simulink model "GFM_NN_closedloop"  (R2025a)
settings: Solver=FixedStepAuto  StartTime=0.0  StopTime=8  FixedStep=1e-6  RelTol=1e-5
PostLoadFcn:
  | , if any(exist('dsrtsu_mdlpostloadfcn', 'file') == [2, 3, 6]), try dsrtsu_mdlpostloadfcn('Execute', bdroot); catch fprintf('Error in PostLoadFcn (dsrtsu_mdlpostloadfcn) for model "%s":\n %s\n', bdroot, lasterr); end, end,
InitFcn:
  | %% ---------sampling time---------
  | fs=10000;
  | Ts = 1/fs; % 1/fs = sampling period;
  | Tsp=Ts;
  | ws=2*pi*fs;
  | Tc = Ts/1;
  | Tch = inf;
  | % Interrupt shift
  | %Tint=0.25e-6;
  | Tint=0.25e-6;
  | %Tint=0;
  | 
  | %% Frequency
  | fsw = 10e3;
  | Tsp = 1 / fsw;
  | % Ts = 1e-6;
  | 
  | %% Grid parameters
  | Vg_LG_RMS = 110;
  | Vg_LL_RMS = Vg_LG_RMS * sqrt(3);
  | f1 = 50;
  | w1 = f1 * 2 * pi;
  | 
  | Lg = 15e-3;
  | Rg = w1 * Lg * 0.05;
  | 
  | %% GFM converter
  | peak_phase_to_earth = sqrt(2)/sqrt(3);
  | SN_GFM = 4e3;
  | PN_GFM = SN_GFM;
  | Vtr_1 = 132;
  | V_base_GFL = Vtr_1*peak_phase_to_earth;
  | I_base_GFL = SN_GFM*peak_phase_to_earth/Vtr_1;
  | 
  | Vs_LL_RMS = Vg_LL_RMS;
  | VDC = 600;
  | 
  | Ls = 3e-3;
  | Rs = w1 * Ls * 0.05;
  | % Rs = 1e-1;
  | Cf = 10e-6;
  | Rf = 1e-3;
  | % Rf = 1;
  | 
  | %% Base values
  | w_Base = 1;
  | %w_Base = 2*pi*f1;
  | V_Base_GFM = sqrt(2) * Vs_LL_RMS / sqrt(3);      % Peak value
  | S_Base_GFM = SN_GFM;
  | I_Base_GFM = sqrt(2) * (S_Base_GFM / 3) / (V_Base_GFM / sqrt(2));     % Peak value
  | Z_Base_GFM = V_Base_GFM / I_Base_GFM;
  | L_Base_GFM = Z_Base_GFM / w_Base;
  | C_Base_GFM = 1 / (w_Base * Z_Base_GFM);
  | 
  | w1_pu = w1 / w_Base;
  | 
  | %% PU values
  | Ls * w1_pu / Z_Base_GFM
  | Ls_pu = Ls / Z_Base_GFM;
  | Lg_pu = Lg / Z_Base_GFM;
  | ... (+142 lines)
model workspace (MAT data in the model file):
  W1 = [0.530351698399 -0.46726077795 -0.189978018403 0.581505596638 -0.976636350155 0.285457074642 -0.344555467367 -0.823834598064 0.260987460613 -0.174824804068 0.166140690446 -2.19062757492 ... (5120 elements, 64x80)]
  W2 = [0.0236483272165 -0.12587569654 -3.47338819504 -0.292541116476 -0.164569035172 -0.37011295557 -0.0788608714938 -0.34808665514 -0.0821482911706 0.0780714154243 -0.721733689308 -0.485419809818 ... (1024 elements, 16x64)]
  W3 = [-0.129827529192 0.112917125225 -0.211720749736 0.109386667609 -1.40702748299 -1.11484694481 -0.318361610174 0.218052342534 0.374470740557 -0.190498560667 -0.238774597645 0.996348917484 ... (16 elements, 1x16)]
  b1 = [-8.9806804657 -10.8322944641 0.357735663652 -8.11319255829 -12.3089160919 -6.15159845352 -0.239361956716 -10.1425418854 -3.17705559731 -9.53854560852 -2.29398417473 -11.1701593399 ... (64 elements, 64x1)]
  b2 = [-0.136206507683 -0.45766967535 -1.54362010956 -0.556495547295 -0.369174063206 -1.49981951714 -1.85871458054 -0.587826907635 -4.87963867188 -1.14077246189 -0.44449698925 -0.9487388134 ... (16 elements, 16x1)]
  b3 = 2.70423817635
  iqrValues = [999.929682567 999.948806394 999.974126382 1163.68199033 1249.86143465 1016.10909761 999.955656405 999.968539404 999.977085124 999.966554003 999.979581889 999.988183479 ... (80 elements, 1x80)]
  medianValues = [1999.66013382 1999.76293028 1999.73262567 1999.76378275 1999.76361619 1999.77040731 1999.79192245 1999.85691047 1999.87382515 1999.88874694 1999.91524435 1999.91351393 ... (80 elements, 1x80)]
  mu = [-0.108593781339 -0.147308811259 -0.175534555128 -0.136585928467 -0.119784171193 -0.170883245612 -0.185899506459 -0.135931465846 -0.0891217813808 -0.0659545740614 -0.0558679902038 -0.052863332895 ... (80 elements, 1x80)]
  net2 : dlnetwork (value not decoded)
  sigma = [0.7187830922 0.834238393845 0.919900139685 0.688758980318 0.599693957155 0.858339742411 0.965167977116 0.792700626358 0.681503940515 0.658236278259 0.655707879722 0.655775233832 ... (80 elements, 1x80)]
undefined symbols (not defined in the file): DiscIntNeverNeededParam
libraries: spsSeriesRLCBranchLib x18, spsCurrentMeasurementLib x9, simulink x6, spsVoltageMeasurementLib x6, simulink_extras x4, spsGroundLib x4, plecslib_extras x2, deeplib x1, spsDCVoltageSourceLib x1, spsThreePhaseProgrammableVoltageSourceLib x1, spsTwoLevelConverterLib x1, spspowerguiLib x1
(part 2 of 3)

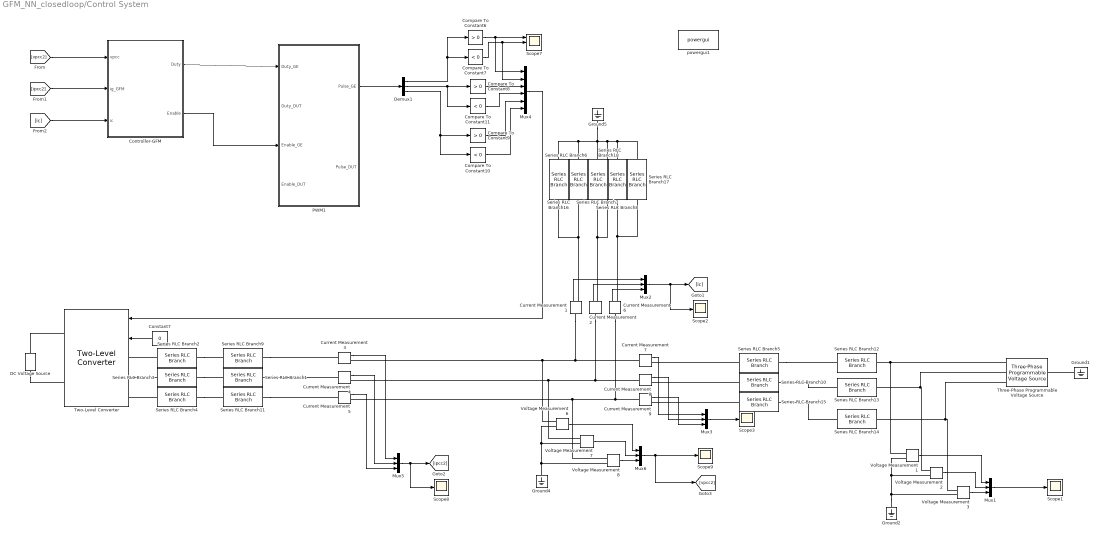
== system GFM_NN_closedloop/Control System ==
  Compare To Constant10 : simulink/Logic and Bit Operations/Compare To Constant  relop=<  const=0  OutDataTypeStr=uint8
  Compare To Constant11 : simulink/Logic and Bit Operations/Compare To Constant  relop=<  const=0  OutDataTypeStr=uint8
  Compare To Constant6 : simulink/Logic and Bit Operations/Compare To Constant  relop=>  const=0  OutDataTypeStr=uint8
  Compare To Constant7 : simulink/Logic and Bit Operations/Compare To Constant  relop=<  const=0  OutDataTypeStr=uint8
  Compare To Constant8 : simulink/Logic and Bit Operations/Compare To Constant  relop=>  const=0  OutDataTypeStr=uint8
  Compare To Constant9 : simulink/Logic and Bit Operations/Compare To Constant  relop=>  const=0  OutDataTypeStr=uint8
  Constant7 : Constant  Value=0
  Controller-GFM : Subsystem
  Current Measurement{1..9} (9 alike) : spsCurrentMeasurementLib/Current Measurement  PhasorSimulation=off  OutputType=Complex  PSBequivalent=0
  DC Voltage Source : spsDCVoltageSourceLib/DC Voltage Source  Amplitude=600  Measurements=None
  Demux1 : Demux  Outputs=3
  Ground{1..2,4..5} (4 alike) : spsGroundLib/Ground  LConnTagsString=a
  Mux{1..3,5..6} (5 alike) : Mux  Inputs=3
  Mux4 : Mux  Inputs=6
  PWM1 : Subsystem
  Scope{1..3,8..9} (5 alike) : Scope
      Scope1 settings: ActiveDisplayYMinimum=-125  ActiveDisplayYMaximum=125
      Scope2 settings: ActiveDisplayYMinimum=-50.45124  ActiveDisplayYMaximum=47.16333
      Scope3 settings: ActiveDisplayYMinimum=-17.02928  ActiveDisplayYMaximum=18.03944  DataLoggingVariableName=Ipcc_f
      Scope8 settings: ActiveDisplayYMinimum=-37.50909  ActiveDisplayYMaximum=37.34562  DataLoggingVariableName=Ipcc
      Scope9 settings: ActiveDisplayYMinimum=-922.38426  ActiveDisplayYMaximum=758.14145
  Scope7 : Scope  NumInputPorts=3
      settings: ActiveDisplayYMinimum=-0.03656  ActiveDisplayYMaximum=1.05589  DataLoggingVariableName=ScopeData2
  Series RLC Branch1 : spsSeriesRLCBranchLib/Series RLC Branch  LConnTagsString=__new0  RConnTagsString=__new0  BranchType=L  Resistance=0.5  Inductance=2e-3  SetiL0=off  InitialCurrent=0  Capacitance=1e-6  Setx0=off  InitialVoltage=0  Measurements=None
  Series RLC Branch{2..5,10,15} (6 alike) : spsSeriesRLCBranchLib/Series RLC Branch  LConnTagsString=__new0  RConnTagsString=__new0  BranchType=R  Resistance=0.2  Inductance=2e-3  SetiL0=off  InitialCurrent=0  Capacitance=1e-6  Setx0=off  InitialVoltage=0  Measurements=None
  Series RLC Branch11 : spsSeriesRLCBranchLib/Series RLC Branch  LConnTagsString=__new0  RConnTagsString=__new0  BranchType=L  Resistance=0.5  Inductance=2e-3  SetiL0=off  InitialCurrent=0  Capacitance=1e-6  Setx0=off  InitialVoltage=0  Measurements=None
  Series RLC Branch12 : spsSeriesRLCBranchLib/Series RLC Branch  LConnTagsString=__new0  RConnTagsString=__new0  BranchType=L  Resistance=0.5  Inductance=20e-3  SetiL0=off  InitialCurrent=0  Capacitance=1e-6  Setx0=off  InitialVoltage=0  Measurements=None
  Series RLC Branch13 : spsSeriesRLCBranchLib/Series RLC Branch  LConnTagsString=__new0  RConnTagsString=__new0  BranchType=L  Resistance=0.5  Inductance=20e-3  SetiL0=off  InitialCurrent=0  Capacitance=1e-6  Setx0=off  InitialVoltage=0  Measurements=None
  Series RLC Branch14 : spsSeriesRLCBranchLib/Series RLC Branch  LConnTagsString=__new0  RConnTagsString=__new0  BranchType=L  Resistance=0.5  Inductance=20e-3  SetiL0=off  InitialCurrent=0  Capacitance=1e-6  Setx0=off  InitialVoltage=0  Measurements=None
  Series RLC Branch16 : spsSeriesRLCBranchLib/Series RLC Branch  LConnTagsString=__new0  RConnTagsString=__new0  BranchType=R  Resistance=20  Inductance=2e-3  SetiL0=off  InitialCurrent=0  Capacitance=1e-6  Setx0=off  InitialVoltage=0  Measurements=None
  Series RLC Branch17 : spsSeriesRLCBranchLib/Series RLC Branch  LConnTagsString=__new0  RConnTagsString=__new0  BranchType=R  Resistance=20  Inductance=2e-3  SetiL0=off  InitialCurrent=0  Capacitance=1e-6  Setx0=off  InitialVoltage=0  Measurements=None
  Series RLC Branch18 : spsSeriesRLCBranchLib/Series RLC Branch  LConnTagsString=__new0  RConnTagsString=__new0  BranchType=R  Resistance=20  Inductance=2e-3  SetiL0=off  InitialCurrent=0  Capacitance=1e-6  Setx0=off  InitialVoltage=0  Measurements=None
  Series RLC Branch6 : spsSeriesRLCBranchLib/Series RLC Branch  LConnTagsString=__new0  RConnTagsString=__new0  BranchType=C  Resistance=0.5  Inductance=5e-3  SetiL0=off  InitialCurrent=0  Capacitance=10e-6  Setx0=off  InitialVoltage=0  Measurements=None
  Series RLC Branch7 : spsSeriesRLCBranchLib/Series RLC Branch  LConnTagsString=__new0  RConnTagsString=__new0  BranchType=C  Resistance=0.5  Inductance=5e-3  SetiL0=off  InitialCurrent=0  Capacitance=10e-6  Setx0=off  InitialVoltage=0  Measurements=None
  Series RLC Branch8 : spsSeriesRLCBranchLib/Series RLC Branch  LConnTagsString=__new0  RConnTagsString=__new0  BranchType=C  Resistance=0.5  Inductance=5e-3  SetiL0=off  InitialCurrent=0  Capacitance=10e-6  Setx0=off  InitialVoltage=0  Measurements=None
  Series RLC Branch9 : spsSeriesRLCBranchLib/Series RLC Branch  LConnTagsString=__new0  RConnTagsString=__new0  BranchType=L  Resistance=0.5  Inductance=2e-3  SetiL0=off  InitialCurrent=0  Capacitance=1e-6  Setx0=off  InitialVoltage=0  Measurements=None
  Three-Phase Programmable Voltage Source : spsThreePhaseProgrammableVoltageSourceLib/Three-Phase Programmable Voltage Source  PositiveSequence="[100*sqrt(3)/sqrt(2)  0 50]"  VariationEntity=Amplitude  VariationType=Table of time-amplitude pairs  VariationTypeAlt=Step  VariationStep=0.5  VariationRate=10  VariationMagnitude=0.3  VariationFrequency=2  VariationTiming=[1 2]  VariationPhaseA=off  Amplitudes=[1 0.5]  TimeValues=[0 5]  HarmonicGeneration=off  HarmonicA=[3 0.2 -25 0]  HarmonicB=[2 0.15 35 2]  Timing="[0.05  3]"  BusType=swing  Pref=0  Qref=0  Qmin=-inf  Qmax=inf
  Two-Level Converter : spsTwoLevelConverterLib/Two-Level Converter  ModelType=Switching devices  Ron=1e-3  Rs=1e6  Cs=inf  Vforward=[0,0]  Ron_Diode=1e-3  Rs_Diode=1e6  Cs_Diode=inf  Vf_Diode=1e-3  Rs_CurrentSource=inf  Ron_ACsource=1e-3
      settings: LibrarySourceBlock=sps_lib/Power Electronics/Two-Level Converter
  Voltage Measurement{1..3,6..8} (6 alike) : spsVoltageMeasurementLib/Voltage Measurement  PhasorSimulation=off  OutputType=Complex  PSBequivalent=0
  powergui1 : spspowerguiLib/powergui  Priority=1  SimulationMode=Discrete  SampleTime=1e-6  frequency=60  Iterations=50  frequencyindice=0  Pbase=100e6  ErrMax=1e-4  UnitsV=kV  UnitsW=MW  buscounter=0  FunctionMessages=off  echomessages=off  EnableUseOfTLC=off  CurrentSourceSwitches=off  DisableSnubberDevices=off  DisableRonSwitches=off  DisableVfSwitches=off  DisplayEquations=off  AutomaticDiscreteSolvers=off  SolverType=Tustin/Backward Euler (TBE)  Interpol=off  ExternalGateDelay=off  methode=off  Ts=100  x0status=blocks  SPID=on  SwTol=0  HookPort=off  NonlinearTolerance=1e-4  nMaxIteration=100  ContinueOnMaxIteration=off  RestoreLinks=warning  ResistiveCurrentMeasurement=off  Frange=[0:2:500]  Ylog=off  Xlog=on  ShowGrid=off  save=off  variable=ZData  structure=0  ZoomFFT=off  StartTime=0.0  cycles=1  DisplayStyle=1  fundamental=60  FreqAxis=off  MaxFrequency=1000  frequencyindicesteady=1  RmsSteady=1  display=off
  wires:
  Mux4/1 -> Two-Level Converter/1
  Constant7/1 -> Two-Level Converter/2
  Compare To Constant7/1 -> Mux4/2, Scope7/2
  PWM1/1(Pulse_GE) -> Demux1/1
  Compare To Constant9/1 -> Mux4/5
  Compare To Constant11/1 -> Mux4/4
  Compare To Constant6/1 -> Scope7/1, Mux4/1
  Demux1/3 -> Compare To Constant10/1, Compare To Constant9/1
  Demux1/1 -> Compare To Constant7/1, Compare To Constant6/1
  Compare To Constant8/1 -> Mux4/3
  Demux1/2 -> Compare To Constant11/1, Compare To Constant8/1
  Compare To Constant10/1 -> Mux4/6
  Current Measurement3/1 -> Mux5/1
  Current Measurement4/1 -> Mux5/2
  Current Measurement5/1 -> Mux5/3
  Voltage Measurement7/1 -> Mux6/2
  Voltage Measurement6/1 -> Mux6/1
  Mux6/1 -> [vpcc2], Scope9/1
  Voltage Measurement8/1 -> Mux6/3
  Current Measurement7/1 -> Mux3/1
  Current Measurement8/1 -> Mux3/2
  Current Measurement9/1 -> Mux3/3
  Mux3/1 -> Scope3/1
  Mux5/1 -> Scope8/1, [ipcc2]
  Mux1/1 -> Scope1/1
  Voltage Measurement3/1 -> Mux1/3
  Voltage Measurement1/1 -> Mux1/1
  Voltage Measurement2/1 -> Mux1/2
  [vpcc2] -> Controller-GFM/1(vpcc)
  [ipcc2] -> Controller-GFM/2(ig_GFM)
  Controller-GFM/1(Duty) -> PWM1/1(Duty_GE)
  Controller-GFM/2(Enable) -> PWM1/3(Enable_GE)
  Current Measurement1/1 -> Mux2/1
  Current Measurement2/1 -> Mux2/2
  Current Measurement6/1 -> Mux2/3
  Mux2/1 -> Scope2/1, [ic]
  [ic] -> Controller-GFM/3(ic)
  connections:
  DC Voltage Source/RConn1 -- Two-Level Converter/RConn1
  DC Voltage Source/LConn1 -- Two-Level Converter/RConn2
  Series RLC Branch11/RConn1 -- Current Measurement5/LConn1
  Series RLC Branch1/RConn1 -- Current Measurement4/LConn1
  Series RLC Branch9/RConn1 -- Current Measurement3/LConn1
  Voltage Measurement7/LConn2 -- Voltage Measurement6/LConn2 -- Voltage Measurement8/LConn2 -- Ground4/LConn1
  Voltage Measurement7/LConn1 -- Current Measurement2/LConn1 -- Current Measurement8/LConn1 -- Current Measurement4/RConn1
  Series RLC Branch6/LConn1 -- Series RLC Branch16/LConn1 -- Series RLC Branch17/LConn1 -- Series RLC Branch8/LConn1 -- Series RLC Branch18/LConn1 -- Ground5/LConn1 -- Series RLC Branch7/LConn1
  Current Measurement3/RConn1 -- Current Measurement1/LConn1 -- Current Measurement7/LConn1 -- Voltage Measurement6/LConn1
  Current Measurement5/RConn1 -- Current Measurement6/LConn1 -- Current Measurement9/LConn1 -- Voltage Measurement8/LConn1
  Voltage Measurement1/LConn1 -- Series RLC Branch12/RConn1 -- Three-Phase Programmable Voltage Source/RConn1
  Voltage Measurement2/LConn1 -- Three-Phase Programmable Voltage Source/RConn2 -- Series RLC Branch13/RConn1
  Voltage Measurement3/LConn1 -- Three-Phase Programmable Voltage Source/RConn3 -- Series RLC Branch14/RConn1
  Ground1/LConn1 -- Three-Phase Programmable Voltage Source/LConn1
  Ground2/LConn1 -- Voltage Measurement3/LConn2 -- Voltage Measurement2/LConn2 -- Voltage Measurement1/LConn2
  Series RLC Branch2/LConn1 -- Two-Level Converter/LConn1
  Series RLC Branch2/RConn1 -- Series RLC Branch9/LConn1
  Series RLC Branch3/LConn1 -- Two-Level Converter/LConn2
  Series RLC Branch3/RConn1 -- Series RLC Branch1/LConn1
  Series RLC Branch4/LConn1 -- Two-Level Converter/LConn3
  Series RLC Branch4/RConn1 -- Series RLC Branch11/LConn1
  Series RLC Branch5/RConn1 -- Series RLC Branch12/LConn1
  Series RLC Branch5/LConn1 -- Current Measurement7/RConn1
  Series RLC Branch10/LConn1 -- Current Measurement8/RConn1
  Series RLC Branch10/RConn1 -- Series RLC Branch13/LConn1
  Series RLC Branch15/LConn1 -- Current Measurement9/RConn1
  Series RLC Branch15/RConn1 -- Series RLC Branch14/LConn1
  Current Measurement1/RConn1 -- Series RLC Branch16/RConn1 -- Series RLC Branch6/RConn1
  Series RLC Branch7/RConn1 -- Series RLC Branch18/RConn1 -- Current Measurement2/RConn1
  Series RLC Branch8/RConn1 -- Series RLC Branch17/RConn1 -- Current Measurement6/RConn1

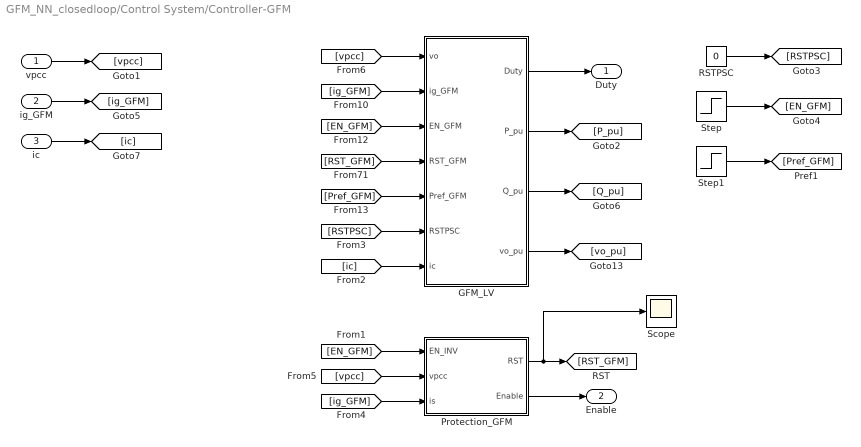
== system GFM_NN_closedloop/Control System/Controller-GFM ==
  vpcc : Inport
  ig_GFM : Inport  Port=2
  ic : Inport  Port=3
  GFM_LV : Subsystem
  Protection_GFM : Subsystem
  RSTPSC : Constant  Value=0
  Scope : Scope
      settings: ActiveDisplayYMinimum=-0.125  ActiveDisplayYMaximum=1.125  DataLoggingVariableName=ScopeData3
  Step : Step  Time=0.5  SampleTime=0
  Step1 : Step  Time=3  After=1500  SampleTime=0
  Duty : Outport  VectorParamsAs1DForOutWhenUnconnected=off
  Enable : Outport  Port=2  VectorParamsAs1DForOutWhenUnconnected=off
  wires:
  vpcc/1 -> [vpcc]
  ig_GFM/1 -> [ig_GFM]
  [vpcc] -> GFM_LV/1(vo)
  [ig_GFM] -> GFM_LV/2(ig_GFM)
  [EN_GFM] -> GFM_LV/3(EN_GFM)
  [Pref_GFM] -> GFM_LV/5(Pref_GFM)
  GFM_LV/2(P_pu) -> [P_pu]
  GFM_LV/3(Q_pu) -> [Q_pu]
  GFM_LV/1(Duty) -> Duty/1
  [EN_GFM] -> Protection_GFM/1(EN_INV)
  Protection_GFM/1(RST) -> Scope/1, [RST_GFM]
  Protection_GFM/2(Enable) -> Enable/1
  [ig_GFM] -> Protection_GFM/3(is)
  [vpcc] -> Protection_GFM/2(vpcc)
  Step/1 -> [EN_GFM]
  RSTPSC/1 -> [RSTPSC]
  Step1/1 -> [Pref_GFM]
  GFM_LV/4(vo_pu) -> [vo_pu]
  [RSTPSC] -> GFM_LV/6(RSTPSC)
  [RST_GFM] -> GFM_LV/4(RST_GFM)
  ic/1 -> [ic]
  [ic] -> GFM_LV/7(ic)

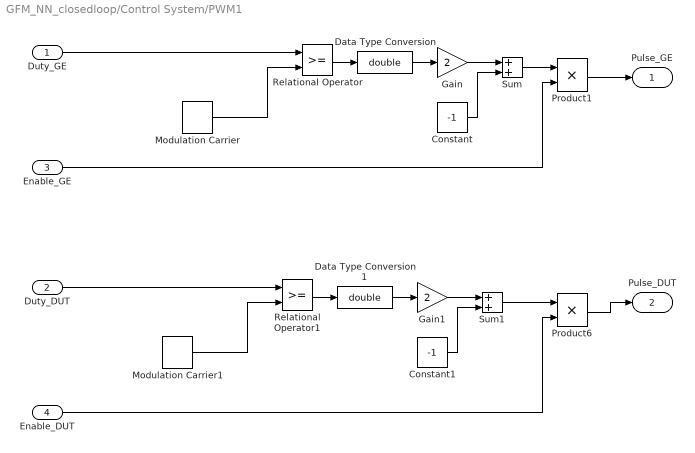
== system GFM_NN_closedloop/Control System/PWM1 ==
  Duty_GE : Inport
  Duty_DUT : Inport  Port=2
  Enable_GE : Inport  Port=3
  Enable_DUT : Inport  Port=4
  Constant : Constant  Value=-1  SampleTime=-1
  Constant1 : Constant  Value=-1  SampleTime=-1
  Data Type Conversion : DataTypeConversion  OutDataTypeStr=double
  Data Type Conversion1 : DataTypeConversion  OutDataTypeStr=double
  Gain : Gain  Gain=2  SaturateOnIntegerOverflow=on  OutDataTypeStr=Inherit: Same as input  ParamDataTypeStr=Inherit: Same as input
  Gain1 : Gain  Gain=2  SaturateOnIntegerOverflow=on  OutDataTypeStr=Inherit: Same as input  ParamDataTypeStr=Inherit: Same as input
  Modulation Carrier : plecslib_extras/Modulators/Symmetrical PWM/Modulation Carrier  fc=10e3  offset=mod(0.5, 1)  range=[0 1]
  Modulation Carrier1 : plecslib_extras/Modulators/Symmetrical PWM/Modulation Carrier  fc=10e3  offset=mod(0.5, 1)  range=[0 1]
  Product1 : Product
  Product6 : Product
  Relational Operator : RelationalOperator
  Relational Operator1 : RelationalOperator
  Sum : Sum  InputSameDT=on  SaturateOnIntegerOverflow=on  OutDataTypeStr=Inherit: Same as first input
  Sum1 : Sum  InputSameDT=on  SaturateOnIntegerOverflow=on  OutDataTypeStr=Inherit: Same as first input
  Pulse_GE : Outport  VectorParamsAs1DForOutWhenUnconnected=off
  Pulse_DUT : Outport  Port=2  VectorParamsAs1DForOutWhenUnconnected=off
  wires:
  Duty_GE/1 -> Relational Operator/1
  Modulation Carrier/1 -> Relational Operator/2
  Relational Operator/1 -> Data Type Conversion/1
  Gain/1 -> Sum/1
  Constant/1 -> Sum/2
  Data Type Conversion/1 -> Gain/1
  Data Type Conversion1/1 -> Gain1/1
  Constant1/1 -> Sum1/2
  Gain1/1 -> Sum1/1
  Relational Operator1/1 -> Data Type Conversion1/1
  Modulation Carrier1/1 -> Relational Operator1/2
  Duty_DUT/1 -> Relational Operator1/1
  Sum1/1 -> Product6/1
  Product6/1 -> Pulse_DUT/1
  Enable_DUT/1 -> Product6/2
  Sum/1 -> Product1/1
  Product1/1 -> Pulse_GE/1
  Enable_GE/1 -> Product1/2

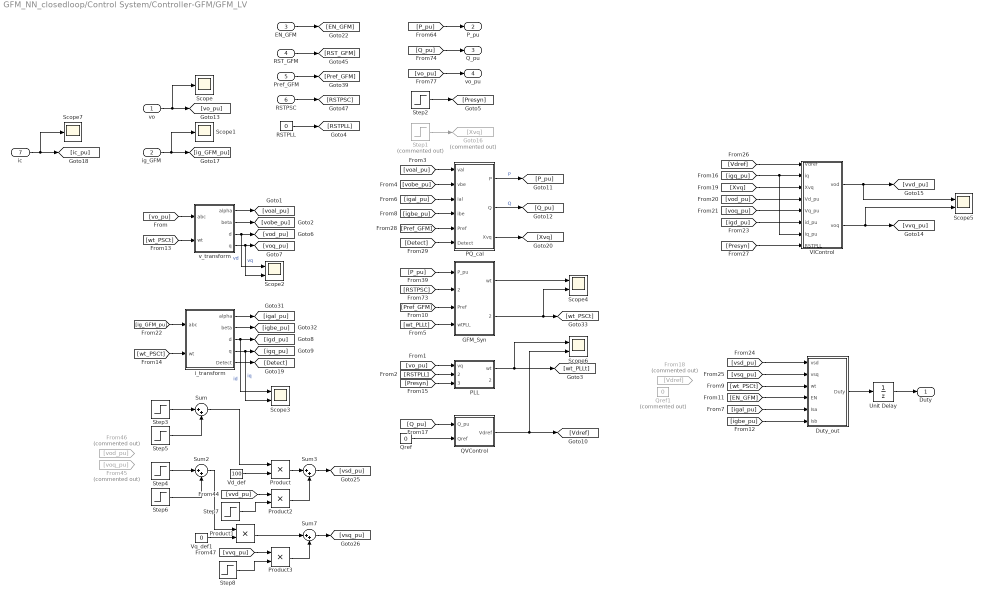
== system GFM_NN_closedloop/Control System/Controller-GFM/GFM_LV ==
  vo : Inport
  ig_GFM : Inport  Port=2
  EN_GFM : Inport  Port=3
  RST_GFM : Inport  Port=4
  Pref_GFM : Inport  Port=5
  RSTPSC : Inport  Port=6
  ic : Inport  Port=7
  Duty_out : Subsystem
  From18 : From  Commented=on  GotoTag=Vdref
  From45 : From  Commented=on  GotoTag=voq_pu
  From46 : From  Commented=on  GotoTag=vod_pu
  GFM_Syn : Subsystem
  Goto16 : Goto  Commented=on  GotoTag=Xvq
  PLL : Subsystem
  PQ_cal : Subsystem
  Product{,1..3} (4 alike) : Product
  QVControl : Subsystem
  Qref : Constant  Value=0
  Qref1 : Constant  Commented=on  Value=0
  RSTPLL : Constant  Value=0
  Scope : Scope
      settings: ActiveDisplayYMinimum=-224.40301  ActiveDisplayYMaximum=188.39301  DataLoggingVariableName=ScopeData4
  Scope1 : Scope
      settings: ActiveDisplayYMinimum=-5.9317  ActiveDisplayYMaximum=5.05503  DataLoggingVariableName=ScopeData5
  Scope{2..6} (5 alike) : Scope  NumInputPorts=2
      Scope2 settings: ActiveDisplayYMinimum=-686.32564  ActiveDisplayYMaximum=654.29928  DataLoggingVariableName=ScopeData9
      Scope3 settings: ActiveDisplayYMinimum=-36.80832  ActiveDisplayYMaximum=81.95422  DataLoggingVariableName=ScopeData10
      Scope4 settings: ActiveDisplayYMinimum=-592.09969  ActiveDisplayYMaximum=5328.89724  DataLoggingVariableName=ScopeData4
      Scope5 settings: ActiveDisplayYMinimum=-140.77704  ActiveDisplayYMaximum=348.97523
      Scope6 settings: ActiveDisplayYMinimum=-35.97431  ActiveDisplayYMaximum=302.6074  DataLoggingVariableName=ScopeData2
  Scope7 : Scope
      settings: ActiveDisplayYMinimum=-5.9317  ActiveDisplayYMaximum=5.05503  DataLoggingVariableName=ScopeData2
  Step1 : Step  Commented=on  Time=5.2  After=0  SampleTime=0
  Step2 : Step  Before=1  After=0  SampleTime=0
  Step3 : Step  Time=1.5  Before=1  After=0.5  SampleTime=0
  Step4 : Step  Time=1.5  Before=1  After=0.5  SampleTime=0
  Step5 : Step  Time=2  After=-0.5  SampleTime=0
  Step6 : Step  Time=2  After=-0.5  SampleTime=0
  Step7 : Step  Time=1.2  SampleTime=0
  Step8 : Step  Time=1.2  SampleTime=0
  Sum{,2..3,7} (4 alike) : Sum  Inputs=|++
  Unit Delay : UnitDelay  SampleTime=Ts  HasFrameUpgradeWarning=on
  VIControl : Subsystem
  Vd_def : Constant  Value=100
  Vq_def1 : Constant  Value=0
  i_transform : Subsystem
  v_transform : Subsystem
  Duty : Outport
  P_pu : Outport  Port=2
  Q_pu : Outport  Port=3
  vo_pu : Outport  Port=4
  wires:
  [voal_pu] -> PQ_cal/1(val)
  [vobe_pu] -> PQ_cal/2(vbe)
  [igal_pu] -> PQ_cal/3(ial)
  [igbe_pu] -> PQ_cal/4(ibe)
  PQ_cal/1(P) -> [P_pu]  "P"
  PQ_cal/2(Q) -> [Q_pu]  "Q"
  EN_GFM/1 -> [EN_GFM]
  [wt_PSCt] -> i_transform/2(wt)
  [ig_GFM_pu] -> i_transform/1(abc)
  [vo_pu] -> v_transform/1(abc)
  [wt_PSCt] -> v_transform/2(wt)
  v_transform/1(alpha) -> [voal_pu]
  [wt_PSCt] -> Duty_out/3(wt)
  [EN_GFM] -> Duty_out/4(EN)
  i_transform/1(alpha) -> [igal_pu]
  i_transform/2(beta) -> [igbe_pu]
  GFM_Syn/1(wt) -> Scope4/1
  [P_pu] -> GFM_Syn/1(P_pu)
  GFM_Syn/2(wtmod) -> Scope4/2, [wt_PSCt]
  RST_GFM/1 -> [RST_GFM]
  [RSTPSC] -> GFM_Syn/2(RSTPSC)
  Pref_GFM/1 -> [Pref_GFM]
  [P_pu] -> P_pu/1
  [Q_pu] -> Q_pu/1
  [vo_pu] -> vo_pu/1
  RSTPSC/1 -> [RSTPSC]
  v_transform/2(beta) -> [vobe_pu]
  [Pref_GFM] -> GFM_Syn/3(Pref)
  Duty_out/1(Duty) -> Unit Delay/1
  Unit Delay/1 -> Duty/1
  [igal_pu] -> Duty_out/5(Isa)
  [igbe_pu] -> Duty_out/6(Isb)
  [RSTPLL] -> PLL/2(RSTPLL)
  [vo_pu] -> PLL/1(vq)
  RSTPLL/1 -> [RSTPLL]
  [wt_PLLt] -> GFM_Syn/4(wtPLL)
  Step2/1 -> [Presyn]
  [Presyn] -> PLL/3(Presyn)
  vo/1 -> Scope/1, [vo_pu]
  ig_GFM/1 -> Scope1/1, [ig_GFM_pu]
  v_transform/3(d) -> Scope2/1, [vod_pu]  "vd"
  v_transform/4(q) -> Scope2/2, [voq_pu]  "vq"
  i_transform/3(d) -> Scope3/1, [igd_pu]  "id"
  i_transform/4(q) -> Scope3/2, [igq_pu]  "iq"
  [Q_pu] -> QVControl/1(Q_pu)
  QVControl/1(Vdref) -> Scope6/2, [Vdref]
  Qref/1 -> QVControl/2(Qref)
  [igq_pu] -> VIControl/7(iq_pu), VIControl/2(iq)
  [Xvq] -> VIControl/3(Xvq)
  [vod_pu] -> VIControl/4(Vd_pu)
  [voq_pu] -> VIControl/5(Vq_pu)
  [igd_pu] -> VIControl/6(id_pu)
  Step1/1 -> Goto16/1
  [Vdref] -> VIControl/1(Vdref)
  PLL/1(wt) -> Scope6/1, [wt_PLLt]
  [Presyn] -> VIControl/8(RSTPLL)
  [vsd_pu] -> Duty_out/1(vsd)
  [vsq_pu] -> Duty_out/2(vsq)
  Step6/1 -> Sum2/2
  Sum2/1 -> Product1/1
  Product1/1 -> Sum7/1
  Step5/1 -> Sum/2
  Product/1 -> Sum3/1
  Sum3/1 -> [vsd_pu]
  Sum/1 -> Product/1
  Step4/1 -> Sum2/1
  Sum7/1 -> [vsq_pu]
  Step3/1 -> Sum/1
  ic/1 -> Scope7/1, [ic_pu]
  VIControl/1(vod) -> [vvd_pu], Scope5/1
  VIControl/2(voq) -> [vvq_pu], Scope5/2
  [Pref_GFM] -> PQ_cal/5(Pref)
  i_transform/5(Detect) -> [Detect]
  [Detect] -> PQ_cal/6(Detect)
  PQ_cal/3(Xvq) -> [Xvq]
  [vvd_pu] -> Product2/1
  Product2/1 -> Sum3/2
  Step7/1 -> Product2/2
  Product3/1 -> Sum7/2
  [vvq_pu] -> Product3/1
  Step8/1 -> Product3/2
  Vd_def/1 -> Product/2
  Vq_def1/1 -> Product1/2

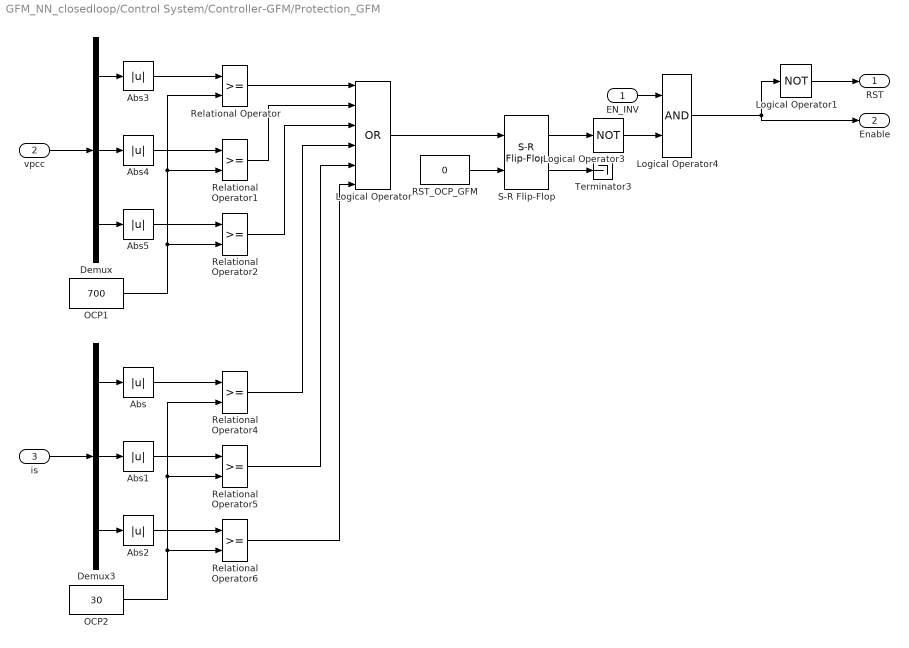
== system GFM_NN_closedloop/Control System/Controller-GFM/Protection_GFM ==
  EN_INV : Inport
  vpcc : Inport  Port=2
  is : Inport  Port=3
  Abs{,1..5} (6 alike) : Abs  SaturateOnIntegerOverflow=off
  Demux : Demux  Outputs=3
  Demux3 : Demux  Outputs=3
  Logical Operator : Logic  Operator=OR  Inputs=6  AllPortsSameDT=off  OutDataTypeStr=boolean
  Logical Operator1 : Logic  Operator=NOT  Inputs=1  IconShape=distinctive  AllPortsSameDT=off  OutDataTypeStr=boolean
  Logical Operator3 : Logic  Operator=NOT  Inputs=1  IconShape=distinctive  AllPortsSameDT=off  OutDataTypeStr=boolean
  Logical Operator4 : Logic  AllPortsSameDT=off  OutDataTypeStr=boolean
  OCP1 : Constant  Value=700
  OCP2 : Constant  Value=30
  RST_OCP_GFM : Constant  Value=0  OutDataTypeStr=boolean  SampleTime=-1
  Relational Operator{,1..2,4..6} (6 alike) : RelationalOperator  OutDataTypeStr=boolean  InputSameDT=off
  S-R Flip-Flop : simulink_extras/Flip Flops/S-R Flip-Flop  initial_condition=0
  Terminator3 : Terminator
  RST : Outport
  Enable : Outport  Port=2
  wires:
  Logical Operator1/1 -> RST/1
  Relational Operator/1 -> Logical Operator/1
  S-R Flip-Flop/1 -> Logical Operator3/1
  Relational Operator2/1 -> Logical Operator/3
  OCP2/1 -> Relational Operator6/2, Relational Operator5/2, Relational Operator4/2
  Relational Operator4/1 -> Logical Operator/4
  Logical Operator3/1 -> Logical Operator4/2
  Relational Operator5/1 -> Logical Operator/5
  Demux/1 -> Abs3/1
  OCP1/1 -> Relational Operator/2, Relational Operator1/2, Relational Operator2/2
  Relational Operator6/1 -> Logical Operator/6
  Demux/2 -> Abs4/1
  RST_OCP_GFM/1 -> S-R Flip-Flop/2
  Demux/3 -> Abs5/1
  S-R Flip-Flop/2 -> Terminator3/1
  Logical Operator/1 -> S-R Flip-Flop/1
  Demux3/1 -> Abs/1
  Demux3/2 -> Abs1/1
  EN_INV/1 -> Logical Operator4/1
  Abs4/1 -> Relational Operator1/1
  Relational Operator1/1 -> Logical Operator/2
  Abs1/1 -> Relational Operator5/1
  Abs3/1 -> Relational Operator/1
  Demux3/3 -> Abs2/1
  Abs/1 -> Relational Operator4/1
  Logical Operator4/1 -> Logical Operator1/1, Enable/1
  Abs2/1 -> Relational Operator6/1
  Abs5/1 -> Relational Operator2/1
  vpcc/1 -> Demux/1
  is/1 -> Demux3/1

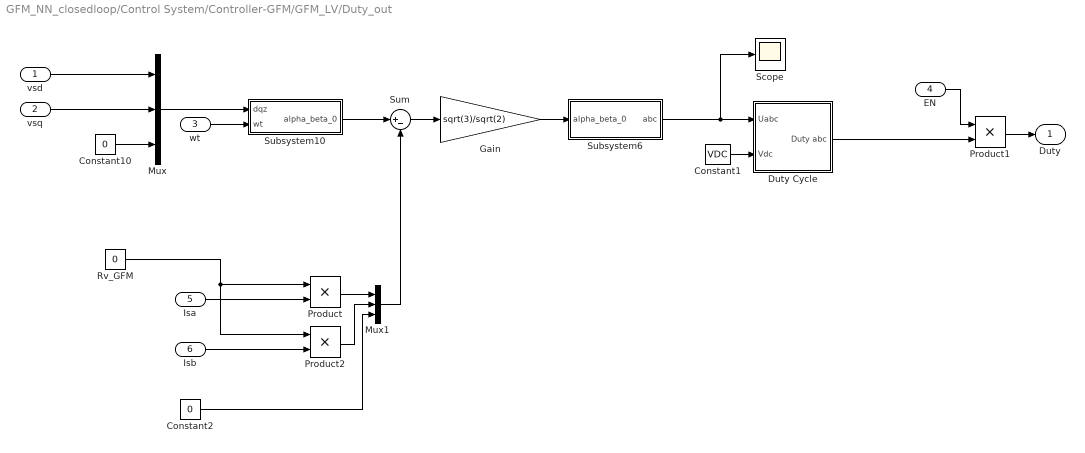
== system GFM_NN_closedloop/Control System/Controller-GFM/GFM_LV/Duty_out ==
  vsd : Inport
  vsq : Inport  Port=2
  wt : Inport  Port=3
  EN : Inport  Port=4
  Isa : Inport  Port=5
  Isb : Inport  Port=6
  Constant1 : Constant  Value=VDC
  Constant10 : Constant  Value=0
  Constant2 : Constant  Value=0
  Duty Cycle : Subsystem
  Gain : Gain  Gain=sqrt(3)/sqrt(2)
  Mux : Mux  Inputs=3
  Mux1 : Mux  Inputs=3
  Product : Product
  Product1 : Product
  Product2 : Product
  Rv_GFM : Constant  Value=0
  Scope : Scope
      settings: ActiveDisplayYMinimum=-202.9779  ActiveDisplayYMaximum=184.85798  DataLoggingVariableName=ScopeData7
  Subsystem10 : Subsystem
  Subsystem6 : Subsystem
  Sum : Sum  Inputs=|+-
  Duty : Outport
  wires:
  Product1/1 -> Duty/1
  Constant10/1 -> Mux/3
  EN/1 -> Product1/1
  Subsystem6/1(abc) -> Scope/1, Duty Cycle/1(Uabc)
  Constant1/1 -> Duty Cycle/2(Vdc)
  Mux/1 -> Subsystem10/1(dqz)
  wt/1 -> Subsystem10/2(wt)
  vsd/1 -> Mux/1
  vsq/1 -> Mux/2
  Duty Cycle/1(Duty abc) -> Product1/2
  Isa/1 -> Product/2
  Isb/1 -> Product2/2
  Rv_GFM/1 -> Product2/1, Product/1
  Subsystem10/1(alpha_beta_0) -> Sum/1
  Product/1 -> Mux1/1
  Product2/1 -> Mux1/2
  Mux1/1 -> Sum/2
  Constant2/1 -> Mux1/3
  Sum/1 -> Gain/1
  Gain/1 -> Subsystem6/1(alpha_beta_0)

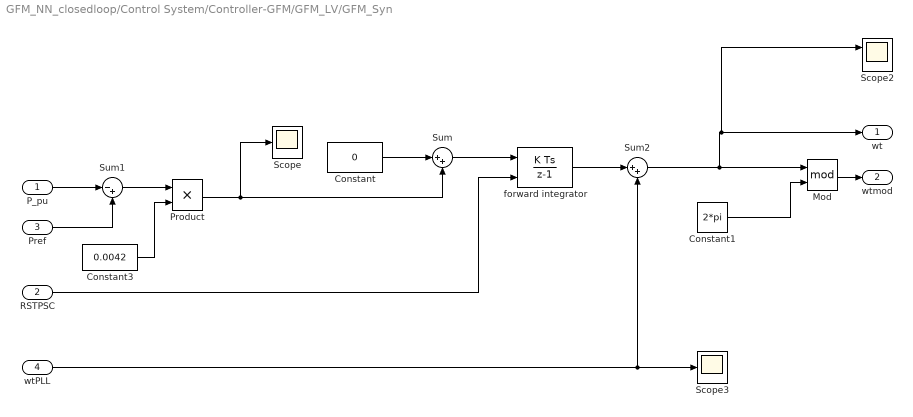
== system GFM_NN_closedloop/Control System/Controller-GFM/GFM_LV/GFM_Syn ==
  P_pu : Inport
  RSTPSC : Inport  Port=2
  Pref : Inport  Port=3
  wtPLL : Inport  Port=4
  Constant : Constant  Value=0
  Constant1 : Constant  Value=2*pi
  Constant3 : Constant  Value=0.0042
  Mod : Math  Operator=mod  SignedPower=on
  Product : Product
  Scope : Scope
      settings: ActiveDisplayYMinimum=-221.44913  ActiveDisplayYMaximum=185.90627  DataLoggingVariableName=ScopeData6
  Scope2 : Scope  NumInputPorts=2
      settings: ActiveDisplayYMinimum=-589.33689  ActiveDisplayYMaximum=5299.63804
  Scope3 : Scope
      settings: ActiveDisplayYMinimum=-51.78258  ActiveDisplayYMaximum=48.72639  DataLoggingVariableName=ScopeData3
  Sum : Sum  Inputs=|++
  Sum1 : Sum  Inputs=|-+
  Sum2 : Sum  Inputs=|++
  forward integrator : DiscreteIntegrator  ExternalReset=level  SampleTime=-1  ICPrevOutput=DiscIntNeverNeededParam  ICPrevScaledInput=DiscIntNeverNeededParam
  wt : Outport
  wtmod : Outport  Port=2
  wires:
  Constant/1 -> Sum/1
  Constant1/1 -> Mod/2
  Mod/1 -> wtmod/1
  Pref/1 -> Sum1/2
  Sum1/1 -> Product/1
  Product/1 -> Sum/2, Scope/1
  Sum/1 -> forward integrator/1
  forward integrator/1 -> Sum2/1
  wtPLL/1 -> Sum2/2, Scope3/1
  Sum2/1 -> Scope2/1, wt/1, Mod/1
  Constant3/1 -> Product/2
  RSTPSC/1 -> forward integrator/2
  P_pu/1 -> Sum1/1

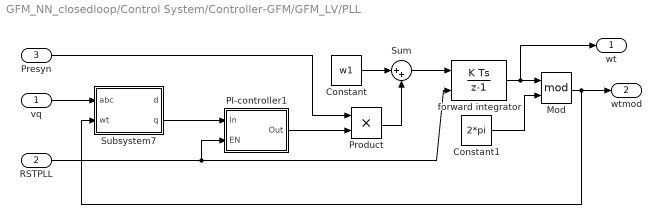
== system GFM_NN_closedloop/Control System/Controller-GFM/GFM_LV/PLL ==
  vq : Inport
  RSTPLL : Inport  Port=2
  Presyn : Inport  Port=3
  Constant : Constant  Value=w1
  Constant1 : Constant  Value=2*pi
  Mod : Math  Operator=mod  SignedPower=on
  PI-controller1 : Subsystem
      mask Display: disp('PI')
  Product : Product
  Subsystem7 : Subsystem
  Sum : Sum  Inputs=|++
  forward integrator : DiscreteIntegrator  ExternalReset=level  SampleTime=-1  ICPrevOutput=DiscIntNeverNeededParam  ICPrevScaledInput=DiscIntNeverNeededParam
  wt : Outport
  wtmod : Outport  Port=2
  wires:
  RSTPLL/1 -> forward integrator/2, PI-controller1/2(EN)
  Sum/1 -> forward integrator/1
  forward integrator/1 -> wt/1, Mod/1
  Constant1/1 -> Mod/2
  Mod/1 -> wtmod/1, Subsystem7/2(wt)
  vq/1 -> Subsystem7/1(abc)
  PI-controller1/1(Out) -> Product/2
  Subsystem7/2(q) -> PI-controller1/1(In)
  Presyn/1 -> Product/1
  Product/1 -> Sum/2
  Constant/1 -> Sum/1

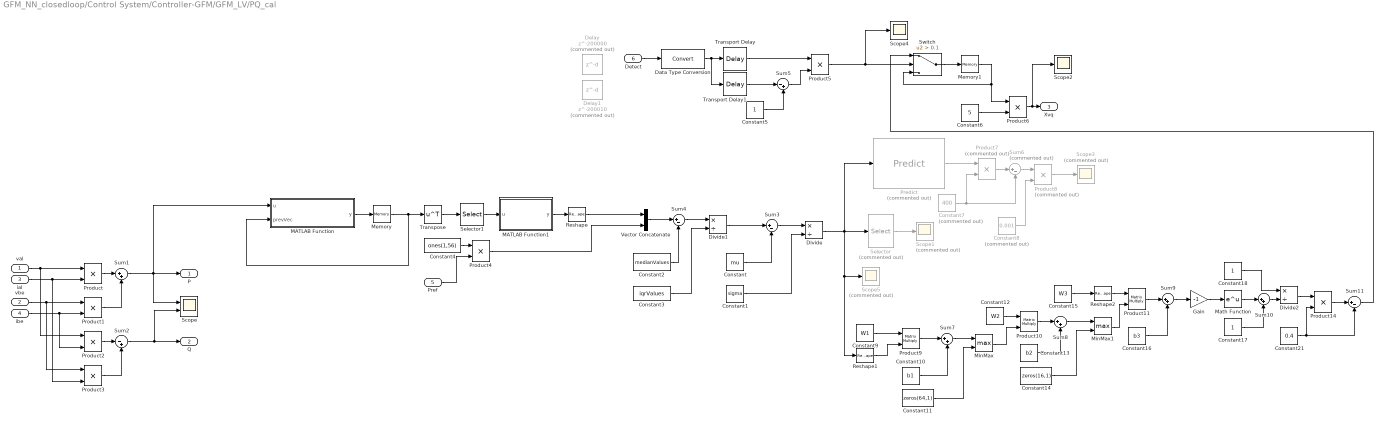
== system GFM_NN_closedloop/Control System/Controller-GFM/GFM_LV/PQ_cal ==
  val : Inport
  vbe : Inport  Port=2
  ial : Inport  Port=3
  ibe : Inport  Port=4
  Pref : Inport  Port=5
  Detect : Inport  Port=6
  Constant : Constant  Value=mu
  Constant1 : Constant  Value=sigma
  Constant10 : Constant  Value=b1
  Constant11 : Constant  Value=zeros(64,1)
  Constant12 : Constant  Value=W2
  Constant13 : Constant  Value=b2
  Constant14 : Constant  Value=zeros(16,1)
  Constant15 : Constant  Value=W3
  Constant16 : Constant  Value=b3
  Constant17 : Constant
  Constant18 : Constant
  Constant2 : Constant  Value=medianValues
  Constant21 : Constant  Value=0.4
  Constant3 : Constant  Value=iqrValues
  Constant4 : Constant  Value=ones(1,56)
  Constant5 : Constant
  Constant6 : Constant  Value=5
  Constant7 : Constant  Commented=on  Value=400
  Constant8 : Constant  Commented=on  Value=0.001
  Constant9 : Constant  Value=W1
  Data Type Conversion : DataTypeConversion  SaturateOnIntegerOverflow=off  RndMeth=Floor
  Delay : Delay  Commented=on  DelayLength=200000  InitialCondition=0
  Delay1 : Delay  Commented=on  DelayLength=200010  InitialCondition=0
  Divide : Product  Inputs=*/
  Divide1 : Product  Inputs=*/
  Divide2 : Product  Inputs=*/
  Gain : Gain  Gain=-1
  MATLAB Function : MATLAB Function  TreatAsAtomicUnit=on
  MATLAB Function1 : MATLAB Function  TreatAsAtomicUnit=on
  Math Function : Math
  Memory : Memory  InitialCondition=zeros(80,1)  InheritSampleTime=on  LinearizeMemory=on  LinearizeAsDelay=on  StateName=statevector
  Memory1 : Memory  InheritSampleTime=on  LinearizeMemory=on  LinearizeAsDelay=on  StateName=statevector
  MinMax : MinMax  Function=max  Inputs=2
  MinMax1 : MinMax  Function=max  Inputs=2
  Predict : deeplib/Predict  Commented=on  Network=Network from MAT-file  NetworkFunction=squeezenet  NetworkFilePath=E:\Research_Aalborg\Backup\Backup\Converter\Transient_fault_location\SimulinkEXP\Transient_model_sim.mat  MiniBatchSize=128  InputDataFormats={'input', 'BC';}  Predictions=on  Activations={}  ForceInterpretedSim=off  EnableDLNetwork=on  LastKnownNetworkFilePath='E:\Research_Aalborg\Backup\Backup\Converter\Transient_fault_location\SimulinkEXP\Transient_model_sim.mat'  LastKnownNetworkTimeStamp=739706.67844907403923571109771728515625
  Product{,1..6,14} (8 alike) : Product
  Product10 : Product  Multiplication=Matrix(*)
  Product11 : Product  Multiplication=Matrix(*)
  Product7 : Product  Commented=on
  Product8 : Product  Commented=on
  Product9 : Product  Multiplication=Matrix(*)
  Reshape : Reshape  OutputDimensionality=Customize  OutputDimensions=[1,24]
  Reshape1 : Reshape  OutputDimensionality=Customize  OutputDimensions=[80,1]
  Reshape2 : Reshape  OutputDimensionality=Customize  OutputDimensions=[1,16]
  Scope : Scope  NumInputPorts=2
      settings: ActiveDisplayYMinimum=-1241.87885  ActiveDisplayYMaximum=6321.54742  DataLoggingVariableName=P_damp
  Scope1 : Scope  Commented=on
      settings: ActiveDisplayYMinimum=-5.34931  ActiveDisplayYMaximum=2.23515  DataLoggingVariableName=P_discrete
  Scope2 : Scope
      settings: ActiveDisplayYMinimum=-2.25  ActiveDisplayYMaximum=0.25  DataLoggingVariableName=Xvq
  Scope3 : Scope  Commented=on
      settings: ActiveDisplayYMinimum=-0.44995  ActiveDisplayYMaximum=0.04958  DataLoggingVariableName=NN_predict
  Scope4 : Scope
      settings: ActiveDisplayYMinimum=-0.125  ActiveDisplayYMaximum=1.125
  Scope5 : Scope  Commented=on
      settings: ActiveDisplayYMinimum=-0.44999  ActiveDisplayYMaximum=0.04991  DataLoggingVariableName=Inputs_NN
  Selector : Selector  Commented=on  InputPortWidth=80  IndexOptions=Index vector (dialog)  Indices=[1 80]  OutputSizes=1
  Selector1 : Selector  InputPortWidth=80  IndexOptions=Index vector (dialog)  Indices=1:24  OutputSizes=24
  Sum{1,7..10} (5 alike) : Sum  Inputs=|++
  Sum11 : Sum  Inputs=|+-
  Sum2 : Sum  Inputs=|-+
  Sum3 : Sum  Inputs=|+-
  Sum4 : Sum  Inputs=|+-
  Sum5 : Sum  Inputs=|-+
  Sum6 : Sum  Commented=on  Inputs=|+-
  Switch : Switch  Criteria=u2 > Threshold  Threshold=0.1  SaturateOnIntegerOverflow=off  InputSameDT=off
  Transport Delay : TransportDelay  DelayTime=0.2
  Transport Delay1 : TransportDelay  DelayTime=0.201
  Transpose : Math  Operator=transpose
  Vector Concatenate : Concatenate
  P : Outport
  Q : Outport  Port=2
  Xvq : Outport  Port=3
  wires:
  vbe/1 -> Product1/1, Product3/1
  Product/1 -> Sum1/1
  Product2/1 -> Sum2/1
  ial/1 -> Product/2, Product3/2
  Product1/1 -> Sum1/2
  val/1 -> Product/1, Product2/1
  Product3/1 -> Sum2/2
  ibe/1 -> Product1/2, Product2/2
  Sum1/1 -> MATLAB Function/1(u), Scope/1, P/1
  Sum2/1 -> Scope/2, Q/1
  MATLAB Function/1(y) -> Memory/1
  Memory/1 -> Transpose/1, MATLAB Function/2(prevVec)
  Selector/1 -> Scope1/1
  Constant/1 -> Sum3/2
  Sum3/1 -> Divide/1
  Constant1/1 -> Divide/2
  Divide/1 -> Predict/1, Reshape1/1, Scope5/1, Selector/1
  Constant3/1 -> Divide1/2
  Constant2/1 -> Sum4/2
  Sum4/1 -> Divide1/1
  Divide1/1 -> Sum3/1
  Constant4/1 -> Product4/1
  Product4/1 -> Vector Concatenate/2
  Pref/1 -> Product4/2
  Vector Concatenate/1 -> Sum4/1
  Transpose/1 -> Selector1/1
  Reshape/1 -> Vector Concatenate/1
  Switch/1 -> Memory1/1
  Memory1/1 -> Product6/1, Switch/3
  Product8/1 -> Scope3/1
  Detect/1 -> Data Type Conversion/1
  Product5/1 -> Scope4/1, Switch/2
  Constant5/1 -> Sum5/2
  Sum5/1 -> Product5/2
  Data Type Conversion/1 -> Transport Delay1/1, Transport Delay/1
  Transport Delay/1 -> Product5/1
  Transport Delay1/1 -> Sum5/1
  Product6/1 -> Scope2/1, Xvq/1
  Constant6/1 -> Product6/2
  Constant7/1 -> Sum6/2, Product7/2
  Product7/1 -> Sum6/1
  Sum6/1 -> Product8/1
  Constant8/1 -> Product8/2
  Selector1/1 -> MATLAB Function1/1(u)
  MATLAB Function1/1(y) -> Reshape/1
  Predict/1 -> Product7/1
  Constant9/1 -> Product9/1
  Reshape1/1 -> Product9/2
  Product9/1 -> Sum7/1
  Constant10/1 -> Sum7/2
  Sum7/1 -> MinMax/1
  Constant11/1 -> MinMax/2
  Constant12/1 -> Product10/1
  MinMax/1 -> Product10/2
  Product10/1 -> Sum8/1
  Constant13/1 -> Sum8/2
  Sum8/1 -> MinMax1/1
  Constant14/1 -> MinMax1/2
  MinMax1/1 -> Product11/2
  Product11/1 -> Sum9/1
  Constant16/1 -> Sum9/2
  Sum9/1 -> Gain/1
  Gain/1 -> Math Function/1
  Math Function/1 -> Sum10/1
  Constant17/1 -> Sum10/2
  Sum10/1 -> Divide2/2
  Constant18/1 -> Divide2/1
  Divide2/1 -> Product14/1
  Constant21/1 -> Sum11/2, Product14/2
  Product14/1 -> Sum11/1
  Sum11/1 -> Switch/1
  Constant15/1 -> Reshape2/1
  Reshape2/1 -> Product11/1

== system GFM_NN_closedloop/Control System/Controller-GFM/GFM_LV/QVControl ==
  Q_pu : Inport
  Qref : Inport  Port=2
  Constant2 : Constant  Value=100
  Constant3 : Constant  Value=0.0033
  Product : Product
  Sum1 : Sum  Inputs=|-+
  Sum2 : Sum  Inputs=|++
  Vdref : Outport
  wires:
  Qref/1 -> Sum1/2
  Sum1/1 -> Product/1
  Constant3/1 -> Product/2
  Product/1 -> Sum2/1
  Constant2/1 -> Sum2/2
  Sum2/1 -> Vdref/1
  Q_pu/1 -> Sum1/1

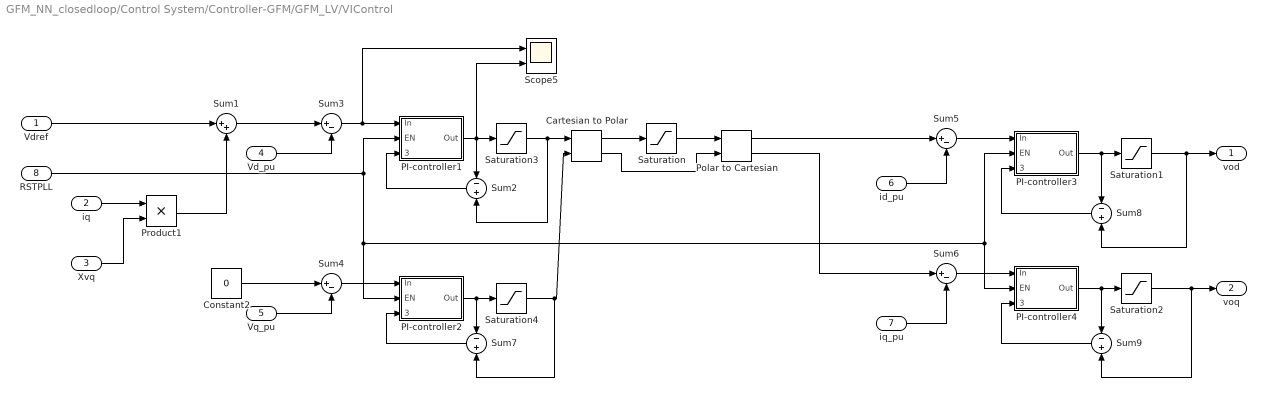
== system GFM_NN_closedloop/Control System/Controller-GFM/GFM_LV/VIControl ==
  Vdref : Inport
  iq : Inport  Port=2
  Xvq : Inport  Port=3
  Vd_pu : Inport  Port=4
  Vq_pu : Inport  Port=5
  id_pu : Inport  Port=6
  iq_pu : Inport  Port=7
  RSTPLL : Inport  Port=8
  Cartesian to Polar : simulink_extras/Transformations/Cartesian to Polar
  Constant2 : Constant  Value=0
  PI-controller1 : Subsystem
      mask Display: disp('PI')
  PI-controller2 : Subsystem
      mask Display: disp('PI')
  PI-controller3 : Subsystem
      mask Display: disp('PI')
  PI-controller4 : Subsystem
      mask Display: disp('PI')
  Polar to Cartesian : simulink_extras/Transformations/Polar to Cartesian
  Product1 : Product
  Saturation : Saturate  UpperLimit=50  LowerLimit=0
  Saturation1 : Saturate  UpperLimit=300  LowerLimit=-300
  Saturation2 : Saturate  UpperLimit=300  LowerLimit=-300
  Saturation3 : Saturate  UpperLimit=100  LowerLimit=-100
  Saturation4 : Saturate  UpperLimit=100  LowerLimit=-100
  Scope5 : Scope  NumInputPorts=2
      settings: ActiveDisplayYMinimum=-272.0155  ActiveDisplayYMaximum=254.97287  DataLoggingVariableName=ScopeData2
  Sum1 : Sum  Inputs=|++
  Sum{2,7..9} (4 alike) : Sum  Inputs=-|+
  Sum{3..6} (4 alike) : Sum  Inputs=|+-
  vod : Outport
  voq : Outport  Port=2
  wires:
  Vdref/1 -> Sum1/1
  iq/1 -> Product1/1
  Xvq/1 -> Product1/2
  Product1/1 -> Sum1/2
  Sum1/1 -> Sum3/1
  Constant2/1 -> Sum4/1
  Sum3/1 -> Scope5/1, PI-controller1/1(In)
  Sum4/1 -> PI-controller2/1(In)
  Sum5/1 -> PI-controller3/1(In)
  Sum6/1 -> PI-controller4/1(In)
  Cartesian to Polar/1 -> Saturation/1
  Saturation/1 -> Polar to Cartesian/1
  Polar to Cartesian/1 -> Sum5/1
  Polar to Cartesian/2 -> Sum6/1
  Cartesian to Polar/2 -> Polar to Cartesian/2
  PI-controller3/1(Out) -> Sum8/1, Saturation1/1
  Saturation1/1 -> Sum8/2, vod/1
  PI-controller4/1(Out) -> Sum9/1, Saturation2/1
  Saturation2/1 -> Sum9/2, voq/1
  RSTPLL/1 -> PI-controller2/2(EN), PI-controller4/2(EN), PI-controller3/2(EN), PI-controller1/2(EN)
  PI-controller1/1(Out) -> Scope5/2, Sum2/1, Saturation3/1
  Saturation3/1 -> Sum2/2, Cartesian to Polar/1
  Sum2/1 -> PI-controller1/3(Windup)
  PI-controller2/1(Out) -> Sum7/1, Saturation4/1
  Saturation4/1 -> Sum7/2, Cartesian to Polar/2
  Sum7/1 -> PI-controller2/3(Windup)
  Sum8/1 -> PI-controller3/3(Windup)
  Sum9/1 -> PI-controller4/3(Windup)
  Vq_pu/1 -> Sum4/2
  Vd_pu/1 -> Sum3/2
  id_pu/1 -> Sum5/2
  iq_pu/1 -> Sum6/2

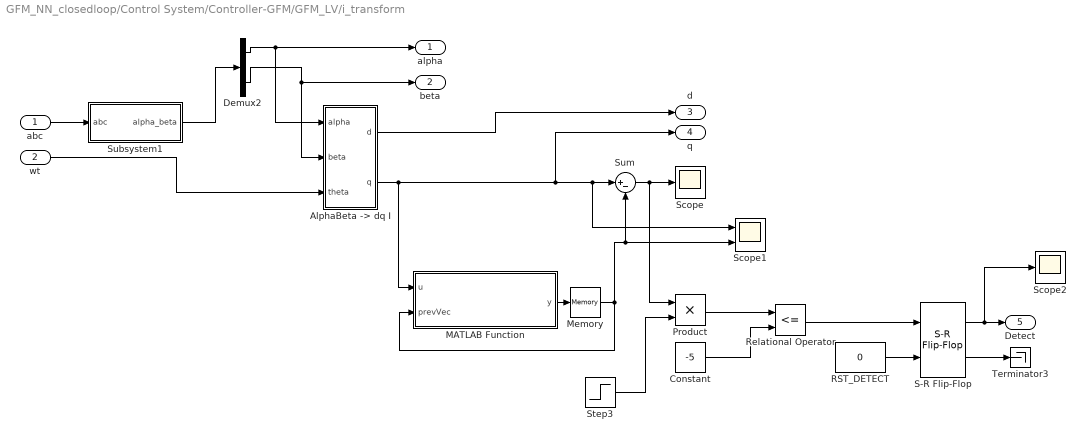
== system GFM_NN_closedloop/Control System/Controller-GFM/GFM_LV/i_transform ==
  abc : Inport
  wt : Inport  Port=2
  "AlphaBeta -> dq I" : Subsystem
  Constant : Constant  Value=-5
  Demux2 : Demux  Outputs=2
  MATLAB Function : MATLAB Function  TreatAsAtomicUnit=on
  Memory : Memory  InheritSampleTime=on  LinearizeMemory=on  LinearizeAsDelay=on
  Product : Product
  RST_DETECT : Constant  Value=0  OutDataTypeStr=boolean  SampleTime=-1
  Relational Operator : RelationalOperator  Operator=<=  OutDataTypeStr=boolean  RndMeth=Simplest  InputSameDT=off
  S-R Flip-Flop : simulink_extras/Flip Flops/S-R Flip-Flop  initial_condition=0
  Scope : Scope
      settings: ActiveDisplayYMinimum=-18.93047  ActiveDisplayYMaximum=29.68165
  Scope1 : Scope  NumInputPorts=2
      settings: ActiveDisplayYMinimum=-26.47465  ActiveDisplayYMaximum=25.16161  DataLoggingVariableName=ScopeData2
  Scope2 : Scope
      settings: ActiveDisplayYMinimum=-0.125  ActiveDisplayYMaximum=1.125  DataLoggingVariableName=Detect_signal
  Step3 : Step  Time=2  SampleTime=0
  Subsystem1 : Subsystem
  Sum : Sum  Inputs=|+-
  Terminator3 : Terminator
  alpha : Outport
  beta : Outport  Port=2
  d : Outport  Port=3
  q : Outport  Port=4
  Detect : Outport  Port=5
  wires:
  Subsystem1/1(alpha_beta) -> Demux2/1
  Demux2/1 -> "AlphaBeta -> dq I"/1(alpha), alpha/1
  Demux2/2 -> "AlphaBeta -> dq I"/2(beta), beta/1
  abc/1 -> Subsystem1/1(abc)
  "AlphaBeta -> dq I"/1(d) -> d/1
  "AlphaBeta -> dq I"/2(q) -> MATLAB Function/1(u), Scope1/1, Sum/1, q/1
  wt/1 -> "AlphaBeta -> dq I"/3(theta)
  Sum/1 -> Product/1, Scope/1
  MATLAB Function/1(y) -> Memory/1
  Memory/1 -> MATLAB Function/2(prevVec), Scope1/2, Sum/2
  Constant/1 -> Relational Operator/2
  Step3/1 -> Product/2
  Product/1 -> Relational Operator/1
  S-R Flip-Flop/2 -> Terminator3/1
  Relational Operator/1 -> S-R Flip-Flop/1
  RST_DETECT/1 -> S-R Flip-Flop/2
  S-R Flip-Flop/1 -> Scope2/1, Detect/1

== system GFM_NN_closedloop/Control System/Controller-GFM/GFM_LV/v_transform ==
  abc : Inport
  wt : Inport  Port=2
  "AlphaBeta -> dq I" : Subsystem
  Demux2 : Demux  Outputs=2
  Subsystem1 : Subsystem
  alpha : Outport
  beta : Outport  Port=2
  d : Outport  Port=3
  q : Outport  Port=4
  wires:
  Subsystem1/1(alpha_beta) -> Demux2/1
  Demux2/1 -> "AlphaBeta -> dq I"/1(alpha), alpha/1
  Demux2/2 -> "AlphaBeta -> dq I"/2(beta), beta/1
  abc/1 -> Subsystem1/1(abc)
  "AlphaBeta -> dq I"/1(d) -> d/1
  "AlphaBeta -> dq I"/2(q) -> q/1
  wt/1 -> "AlphaBeta -> dq I"/3(theta)

== system GFM_NN_closedloop/Control System/Controller-GFM/GFM_LV/Duty_out/Duty Cycle ==
  Uabc : Inport
  Vdc : Inport  Port=2
  Constant2 : Constant  Value=0.5*[1 1 1]
  Product3 : Product  Inputs=*/  SaturateOnIntegerOverflow=on  OutDataTypeStr=Inherit: Same as first input
  Saturation1 : Saturate  UpperLimit=0.98  LowerLimit=0.02
  Saturation4 : Saturate  UpperLimit=1/sqrt(3)  LowerLimit=-1/sqrt(3)
  Sum1 : Sum  Inputs=|++  InputSameDT=on  SaturateOnIntegerOverflow=on  OutDataTypeStr=Inherit: Same as first input
  Duty abc : Outport  VectorParamsAs1DForOutWhenUnconnected=off
  wires:
  Vdc/1 -> Product3/2
  Sum1/1 -> Saturation1/1
  Product3/1 -> Saturation4/1
  Saturation4/1 -> Sum1/1
  Uabc/1 -> Product3/1
  Constant2/1 -> Sum1/2
  Saturation1/1 -> Duty abc/1

== system GFM_NN_closedloop/Control System/Controller-GFM/GFM_LV/Duty_out/Subsystem10 ==
  dqz : Inport
  wt : Inport  Port=2
  Constant : Constant  Value=0
  Demux : Demux  Outputs=3
  Demux1 : Demux  Outputs=2
  Mux : Mux  Inputs=3
  Mux1 : Mux  Inputs=2
  exp(jwT)1 : Subsystem
  alpha_beta_0 : Outport  VectorParamsAs1DForOutWhenUnconnected=off
  wires:
  Mux/1 -> alpha_beta_0/1
  Mux1/1 -> exp(jwT)1/1(dq)
  exp(jwT)1/1(alphabeta) -> Demux1/1
  Demux1/1 -> Mux/1
  dqz/1 -> Demux/1
  Constant/1 -> Mux/3
  Demux/2 -> Mux1/2
  wt/1 -> exp(jwT)1/2(wt)
  Demux/1 -> Mux1/1
  Demux1/2 -> Mux/2

== system GFM_NN_closedloop/Control System/Controller-GFM/GFM_LV/Duty_out/Subsystem6 ==
  alpha_beta_0 : Inport
  Gain1 : Gain  Gain=sqrt(2/3)  SaturateOnIntegerOverflow=on  OutDataTypeStr=Inherit: Same as input  ParamDataTypeStr=Inherit: Same as input
  Gain3 : Gain  Gain="[ 1   0   1/sqrt(2); -1/2   sqrt(3)/2   1/sqrt(2); -1/2  -sqrt(3)/2  1/sqrt(2) ]"  Multiplication=Matrix(K*u) (u vector)  SaturateOnIntegerOverflow=on  OutDataTypeStr=Inherit: Same as input  ParamDataTypeStr=Inherit: Same as input
  abc : Outport  VectorParamsAs1DForOutWhenUnconnected=off
  wires:
  alpha_beta_0/1 -> Gain3/1
  Gain3/1 -> Gain1/1
  Gain1/1 -> abc/1

== system GFM_NN_closedloop/Control System/Controller-GFM/GFM_LV/PLL/PI-controller1 ==
  In : Inport
  EN : Inport  Port=2
  Backward integrator : DiscreteIntegrator  gainval=2  ExternalReset=level  SampleTime=-1  ICPrevOutput=DiscIntNeverNeededParam  ICPrevScaledInput=DiscIntNeverNeededParam
  Gain : Gain
  Sum1 : Sum  SaturateOnIntegerOverflow=on
  Out : Outport  VectorParamsAs1DForOutWhenUnconnected=off
  wires:
  Sum1/1 -> Out/1
  In/1 -> Backward integrator/1, Gain/1  "e(k)"
  Backward integrator/1 -> Sum1/2
  EN/1 -> Backward integrator/2
  Gain/1 -> Sum1/1

== system GFM_NN_closedloop/Control System/Controller-GFM/GFM_LV/PLL/Subsystem7 ==
  abc : Inport
  wt : Inport  Port=2
  "AlphaBeta -> dq I" : Subsystem
  Demux2 : Demux  Outputs=2
  Subsystem1 : Subsystem
  d : Outport
  q : Outport  Port=2
  wires:
  Subsystem1/1(alpha_beta) -> Demux2/1
  Demux2/1 -> "AlphaBeta -> dq I"/1(alpha)
  Demux2/2 -> "AlphaBeta -> dq I"/2(beta)
  abc/1 -> Subsystem1/1(abc)
  "AlphaBeta -> dq I"/1(d) -> d/1
  "AlphaBeta -> dq I"/2(q) -> q/1
  wt/1 -> "AlphaBeta -> dq I"/3(theta)

== system GFM_NN_closedloop/Control System/Controller-GFM/GFM_LV/VIControl/PI-controller1 ==
  In : Inport
  EN : Inport  Port=2
  Windup : Inport  Port=3
  Backward integrator : DiscreteIntegrator  gainval=50  ExternalReset=level  SampleTime=-1  ICPrevOutput=DiscIntNeverNeededParam  ICPrevScaledInput=DiscIntNeverNeededParam
  Product : Product
  Step3 : Step  Time=6  Before=0.1  After=0.1  SampleTime=0
  Sum1 : Sum  SaturateOnIntegerOverflow=on
  Sum2 : Sum  SaturateOnIntegerOverflow=on
  Out : Outport  VectorParamsAs1DForOutWhenUnconnected=off
  wires:
  Sum1/1 -> Out/1
  In/1 -> Product/2, Sum2/1  "e(k)"
  Product/1 -> Sum1/1
  Backward integrator/1 -> Sum1/2
  EN/1 -> Backward integrator/2
  Windup/1 -> Sum2/2
  Sum2/1 -> Backward integrator/1
  Step3/1 -> Product/1

== system GFM_NN_closedloop/Control System/Controller-GFM/GFM_LV/VIControl/PI-controller2 ==
  In : Inport
  EN : Inport  Port=2
  Windup : Inport  Port=3
  Backward integrator : DiscreteIntegrator  gainval=50  ExternalReset=level  SampleTime=-1  ICPrevOutput=DiscIntNeverNeededParam  ICPrevScaledInput=DiscIntNeverNeededParam
  Product : Product
  Step3 : Step  Time=6  Before=0.1  After=0.1  SampleTime=0
  Sum1 : Sum  SaturateOnIntegerOverflow=on
  Sum2 : Sum  SaturateOnIntegerOverflow=on
  Out : Outport  VectorParamsAs1DForOutWhenUnconnected=off
  wires:
  Sum1/1 -> Out/1
  In/1 -> Product/2, Sum2/1  "e(k)"
  Product/1 -> Sum1/1
  Backward integrator/1 -> Sum1/2
  EN/1 -> Backward integrator/2
  Windup/1 -> Sum2/2
  Sum2/1 -> Backward integrator/1
  Step3/1 -> Product/1

== system GFM_NN_closedloop/Control System/Controller-GFM/GFM_LV/VIControl/PI-controller3 ==
  In : Inport
  EN : Inport  Port=2
  Windup : Inport  Port=3
  Backward integrator : DiscreteIntegrator  gainval=12.5  ExternalReset=level  SampleTime=-1  ICPrevOutput=DiscIntNeverNeededParam  ICPrevScaledInput=DiscIntNeverNeededParam
  Gain : Gain  Gain=5
  Sum1 : Sum  SaturateOnIntegerOverflow=on
  Sum2 : Sum  SaturateOnIntegerOverflow=on
  Out : Outport  VectorParamsAs1DForOutWhenUnconnected=off
  wires:
  Sum1/1 -> Out/1
  In/1 -> Sum2/1, Gain/1  "e(k)"
  Gain/1 -> Sum1/1
  Backward integrator/1 -> Sum1/2
  EN/1 -> Backward integrator/2
  Windup/1 -> Sum2/2
  Sum2/1 -> Backward integrator/1

== system GFM_NN_closedloop/Control System/Controller-GFM/GFM_LV/VIControl/PI-controller4 ==
  In : Inport
  EN : Inport  Port=2
  Windup : Inport  Port=3
  Backward integrator : DiscreteIntegrator  gainval=12.5  ExternalReset=level  SampleTime=-1  ICPrevOutput=DiscIntNeverNeededParam  ICPrevScaledInput=DiscIntNeverNeededParam
  Gain : Gain  Gain=5
  Sum1 : Sum  SaturateOnIntegerOverflow=on
  Sum2 : Sum  SaturateOnIntegerOverflow=on
  Out : Outport  VectorParamsAs1DForOutWhenUnconnected=off
  wires:
  Sum1/1 -> Out/1
  In/1 -> Sum2/1, Gain/1  "e(k)"
  Gain/1 -> Sum1/1
  Backward integrator/1 -> Sum1/2
  EN/1 -> Backward integrator/2
  Windup/1 -> Sum2/2
  Sum2/1 -> Backward integrator/1

== system GFM_NN_closedloop/Control System/Controller-GFM/GFM_LV/i_transform/AlphaBeta -> dq I ==
  alpha : Inport
  beta : Inport  Port=2
  theta : Inport  Port=3
  Fcn2 : Fcn  Expr=cos(u(3))*u(1)+sin(u(3))*u(2)
  Fcn3 : Fcn  Expr=-sin(u(3))*u(1)+cos(u(3))*u(2)
  Mux : Mux  Inputs=3
  d : Outport  VectorParamsAs1DForOutWhenUnconnected=off
  q : Outport  Port=2  VectorParamsAs1DForOutWhenUnconnected=off
  wires:
  beta/1 -> Mux/2
  alpha/1 -> Mux/1
  theta/1 -> Mux/3
  Fcn2/1 -> d/1
  Fcn3/1 -> q/1
  Mux/1 -> Fcn3/1, Fcn2/1

== system GFM_NN_closedloop/Control System/Controller-GFM/GFM_LV/i_transform/Subsystem1 ==
  abc : Inport
  Gain1 : Gain  Gain=2/3  SaturateOnIntegerOverflow=on  OutDataTypeStr=Inherit: Same as input  ParamDataTypeStr=Inherit: Same as input
  Gain3 : Gain  Gain="[ 1   -1/2   -1/2; 0   sqrt(3)/2   -sqrt(3)/2]"  Multiplication=Matrix(K*u) (u vector)  SaturateOnIntegerOverflow=on  OutDataTypeStr=Inherit: Same as input  ParamDataTypeStr=Inherit: Same as input
  alpha_beta : Outport  VectorParamsAs1DForOutWhenUnconnected=off
  wires:
  abc/1 -> Gain3/1
  Gain3/1 -> Gain1/1
  Gain1/1 -> alpha_beta/1

== system GFM_NN_closedloop/Control System/Controller-GFM/GFM_LV/v_transform/AlphaBeta -> dq I ==
  alpha : Inport
  beta : Inport  Port=2
  theta : Inport  Port=3
  Fcn2 : Fcn  Expr=cos(u(3))*u(1)+sin(u(3))*u(2)
  Fcn3 : Fcn  Expr=-sin(u(3))*u(1)+cos(u(3))*u(2)
  Mux : Mux  Inputs=3
  d : Outport  VectorParamsAs1DForOutWhenUnconnected=off
  q : Outport  Port=2  VectorParamsAs1DForOutWhenUnconnected=off
  wires:
  beta/1 -> Mux/2
  alpha/1 -> Mux/1
  theta/1 -> Mux/3
  Fcn2/1 -> d/1
  Fcn3/1 -> q/1
  Mux/1 -> Fcn3/1, Fcn2/1

== system GFM_NN_closedloop/Control System/Controller-GFM/GFM_LV/v_transform/Subsystem1 ==
  abc : Inport
  Gain1 : Gain  Gain=2/3  SaturateOnIntegerOverflow=on  OutDataTypeStr=Inherit: Same as input  ParamDataTypeStr=Inherit: Same as input
  Gain3 : Gain  Gain="[ 1   -1/2   -1/2; 0   sqrt(3)/2   -sqrt(3)/2]"  Multiplication=Matrix(K*u) (u vector)  SaturateOnIntegerOverflow=on  OutDataTypeStr=Inherit: Same as input  ParamDataTypeStr=Inherit: Same as input
  alpha_beta : Outport  VectorParamsAs1DForOutWhenUnconnected=off
  wires:
  abc/1 -> Gain3/1
  Gain3/1 -> Gain1/1
  Gain1/1 -> alpha_beta/1
